simulink model "donkeycar_raspi"  (R2021b)
settings: Solver=ode3  StartTime=0.0  StopTime=inf  FixedStep=0.05  RelTol=1e-3  EnableMultiTasking=on
libraries: matrix_library x3, deeplib x1, embedlinuxAVlib x1, raspberrypiAVlib x1
settings Model: FPTRunName=Active  ExtModeTrigDuration=2  Creator=kkoichi  LastModifiedBy=kkoichi
settings SolverCC: AlgebraicLoopSolver=TrustRegion  PositivePriorityOrder=on
settings DataIOCC: LimitDataPoints=on  SaveFormat=Array
settings OptimizationCC: ExpressionDepthLimit=2147483647  ZeroExternalMemoryAtStartup=off  ZeroInternalMemoryAtStartup=off  LifeSpan=Inf  MaxStackSize=64
settings DebuggingCC: UnderspecifiedInitializationDetection=Classic  MergeDetectMultiDrivingBlocksExec=none  FcnCallInpInsideContextMsg=warning  AllowSymbolicDim=off  StateNameClashWarn=warning  SFUnexpectedBacktrackingDiag=warning  SFNoUnconditionalDefaultTransitionDiag=warning  SFExecutionAtInitializationDiag=none  SFMachineParentedDataDiag=warning  ArithmeticOperatorsInVariantConditions=warning
settings HardwareCC: ProdBitPerPointer=32  ProdBitPerSizeT=32  ProdBitPerPtrDiffT=32  ProdLargestAtomicInteger=Long  ProdLargestAtomicFloat=Double  ProdWordSize=32  ProdHWDeviceType=ARM Compatible->ARM Cortex  UseEmbeddedCoderFeatures=off  UseSimulinkCoderFeatures=off
settings ModelReferenceCC: PropagateSignalLabelsOutOfModel=off
settings SFSimCC: SimUseLocalCustomCode=off  CustomCodeUndefinedFunction=UseInterfaceOnly  SimTargetLang=C++
settings RTWCC: Description=Embedded Coder  SystemTargetFile=ert.tlc  HardwareBoard=Raspberry Pi  TLCOptions="-aInlineSetEventsForThisBaseRateFcn=TLC_FALSE -aSuppressMultiTaskScheduler=TLC_FALSE  -aRateBasedStepFcn=0"  TemplateMakefile=ert_default_tmf  GenerateReport=on  RTWVerbose=off  RTWUseLocalCustomCode=off  Toolchain=GNU GCC Embedded Linux  BuildConfiguration=Faster Runs  LaunchReport=on  TargetLang=C++  DLTargetLibrary=arm-compute  DLArmComputeArch=armv8
settings CodeAppCC: ForceParamTrailComments=on  OperatorAnnotations=on  StateflowObjectComments=on  MATLABSourceComments=on
settings ERTTargetCC: TargetLangStandard=C++11 (ISO)  MultiwordLength=2048  ERTCustomFileBanners=off  SupportContinuousTime=on  SupportNonInlinedSFcns=on  RemoveResetFunc=off  SupportVariableSizeSignals=on  ModelStepFunctionPrototypeControlCompliant=off  ExtModeTransport=2  ExtModeStaticAlloc=on  ExtModeMexFile=ext_xcp  ExtModeIntrfLevel=Level2 - Open
settings ConfigComp: CovMetricSettings=dw  CovSaveCumulativeToWorkspaceVar=on  CovSaveSingleToWorkspaceVar=on  CovExternalEMLEnable=off  CovSFcnEnable=off

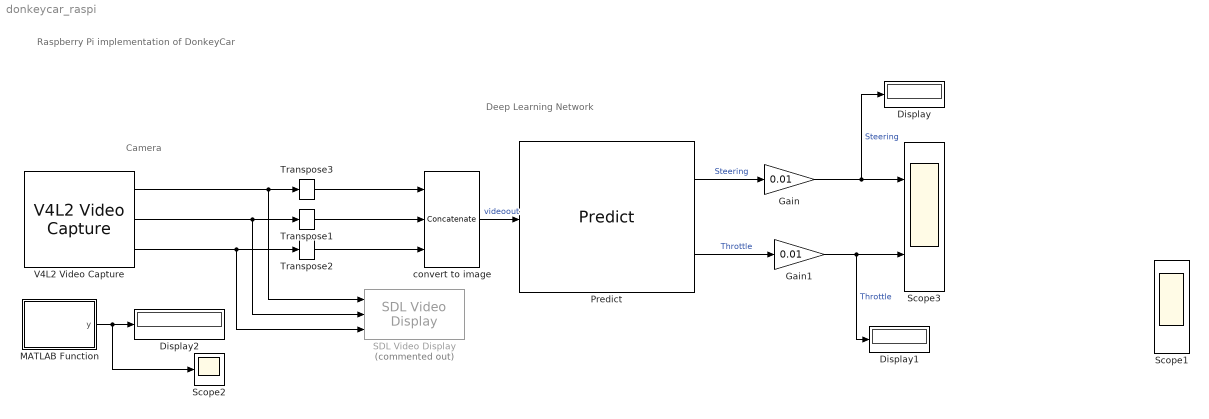
== system donkeycar_raspi ==
  note: Camera
  note: Raspberry Pi implementation of DonkeyCar
  note: Deep Learning Network
  Display : Display
  Display1 : Display
  Display2 : Display
  Gain : Gain  Gain=0.01  OutDataTypeStr=double
  Gain1 : Gain  Gain=0.01  OutDataTypeStr=double
  MATLAB Function : MATLAB Function  TreatAsAtomicUnit=on
  Predict : deeplib/Predict  Network=Network from MAT-file  NetworkFunction=net.mat  NetworkFilePath=C:\data\kkwork\TatamiRacer\MATLAB\donkeyKerasNet.mat  MiniBatchSize=128  InputDataFormats={ '', '' }  Predictions=on  Activations={}  ForceInterpretedSim=off  EnableDLNetwork=on
      settings: SourceProductBaseCode=NN
  SDL Video Display : embedlinuxAVlib/SDL Video Display  Commented=on  title=SDL Video Display  pixelFormat=RGB  pixelOrder=Planar  rowMajor=on  blockPlatform=Raspberry Pi
      settings: SourceProductBaseCode=SC_BEAGLEBONE_BLUE,EMBEDDEDLINUX,NVIDIA,RASPPIIO
  Scope1 : Scope  NumInputPorts=2
  Scope2 : Scope
  Scope3 : Scope  NumInputPorts=2
  Transpose1 : matrix_library/Transpose
      settings: SourceProductBaseCode=SL
  Transpose2 : matrix_library/Transpose
      settings: SourceProductBaseCode=SL
  Transpose3 : matrix_library/Transpose
      settings: SourceProductBaseCode=SL
  V4L2 Video Capture : raspberrypiAVlib/V4L2 Video Capture  DeviceName=/dev/video0  Resolution=160x120  CustomResolution=[120,160]  PixelFormat=RGB  SampleTime=-1  pixelOrder=planar  simOutput=Colorbars  imSizeSelection=320x240  imSize=[640, 480]  roi=[0, 0, 640, 480]  m_devName='/dev/video0'  blockPlatform=LINUX
      settings: SourceProductBaseCode=RASPPI
  convert to image : Concatenate  NumInputs=3  Mode=Multidimensional array  ConcatenateDimension=3
  wires:
  Transpose3/1 -> convert to image/1
  convert to image/1 -> Predict/1  "videoout"
  V4L2 Video Capture/1 -> Transpose3/1, SDL Video Display/1
  V4L2 Video Capture/3 -> SDL Video Display/3, Transpose2/1
  Transpose1/1 -> convert to image/2
  Predict/1 -> Gain/1  "Steering"
  V4L2 Video Capture/2 -> SDL Video Display/2, Transpose1/1
  Predict/2 -> Gain1/1  "Throttle"
  Transpose2/1 -> convert to image/3
  MATLAB Function/1(y) -> Scope2/1, Display2/1
  Gain1/1 -> Display1/1, Scope3/2  "Throttle"
  Gain/1 -> Display/1, Scope3/1  "Steering"

== matlab function donkeycar_raspi/MATLAB Function ==
  data: y output
function y = exec_time()
    persistent t0
    if isempty(t0)
        t0 = 0;
        tic;
    end
    t = toc;
    y = t - t0;
    t0 = t;
end
